simulink model "fm"  (R2023b)
settings: Solver=VariableStepAuto  StartTime=0.0  StopTime=20  RelTol=1e-3
settings Model: Creator=HP  LastModifiedBy=HP

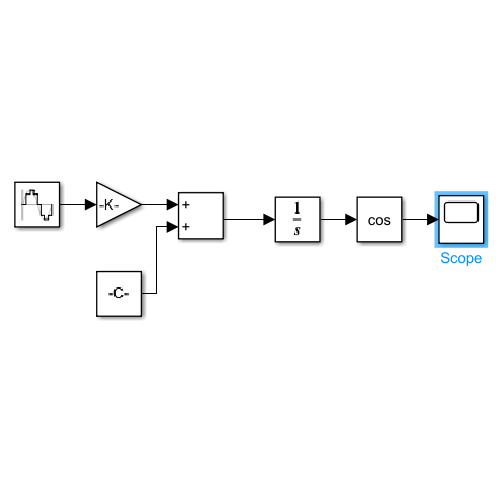
[thumbnail: Simulink's stored preview of the top-level diagram]
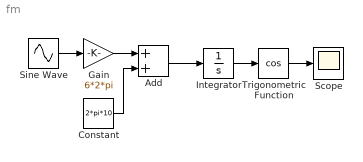
== system fm ==
  Add : Sum
  Constant : Constant  Value=2*pi*10
  Gain : Gain  Gain=6*2*pi
  Integrator : Integrator
  Scope : Scope
  Sine Wave : Sin  Frequency=2*pi  Phase=pi/2  SampleTime=1/5000
  Trigonometric Function : Trigonometry  Operator=cos
  wires:
  Trigonometric Function/1 -> Scope/1
  Integrator/1 -> Trigonometric Function/1
  Add/1 -> Integrator/1
  Gain/1 -> Add/1
  Sine Wave/1 -> Gain/1
  Constant/1 -> Add/2
